simulink model "x35BusNetworkElectricityTransmissionModel"  (R2023b)
settings: Solver=VariableStepAuto  StartTime=0.0  StopTime=0.8  RelTol=1e-3
model workspace (MAT data in the model file):
  Compensation_Ki = 30
  Compensation_Kp = 3
  DC_Ki = 400
  DC_Kp = 8
  F = 0.01
  Flux_min = 0.5
  Grid_Freq_PWM = 2700
  Grid_Ireg_Ki = 5
  Grid_Ireg_Kp = 0.83
  Grid_Ireg_lim = 1.1
  Grid_Modindex_Upper = 1.1
  Grid_conv_Imax = 0.8
  H = 0.685
  Idref_max = 0.9
  Iqref_Tc = 0.3
  Ki_Var = 0.05
  Ki_Vreg = 20
  Ksh = 1.1
  L_pu = 0.3
  Llr = 0.16
  Lls = 0.18
  Lm = 2.9
  Nb_wt = 6
  P_mech = 1080000
  Pitch_Ki = 0
  Pitch_Kp = 150
  Pitch_Max = 27
  Pitch_Tc = 0.01
  Pitch_rate = 10
  Q_Filt = 50
  R_pu = 0.003
  Rotor_Freq_PWM = 1620
  Rotor_Ireg_Ki = 8
  Rotor_Ireg_Kp = 0.6
  Rotor_Ireg_lim = 0.1
  Rotor_Modindex_Upper = 2
  Rr = 0.016
  Rs = 0.023
  T_set = 0.0001
  Tp = 5e-05
  Ts = 5e-06
  Var_C_Filt = 720000
  Var_reg_max = 1.1
  Var_reg_min = 0.9
  WT_Coeff = [0.645 116 0.4 5 21 0.00912 0.08 0.035]
  WT_H = 4.32
  WT_IGBTRon = 5.931
  WT_Param = [91.204 10143]
  Wind_Freq_Filt = 10000
  Wind_Freq_nom = 60
  Wind_P_nom = 1200000
  Wind_Rotor_V_nom = 1950
  Wind_V_nom = 500
  Zeta_Filt = 0.707106781187
  init = [-0.2 0 0 0 0 0 0 0]
  p = 3
  torque0 = 0.83
  v_Ki = 0.1
  v_Kp = 3.6
  v_Max = 1.2
  v_Min = 0.7
  v_T = 5
  vreg_max = 1
  wind_VDC_nom = 1150
  wt0 = 1.2
undefined symbols (not defined in the file): D1, D11, Delta, DiscIntNeverNeededParam, Ion, Lithium, P, Q
libraries: powerlib_extras x144, spsSeriesRLCBranchLib x67, spsLoadFlowBusLib x43, spsThreePhaseTransformerTwoWindingsLib x32, spsThreePhaseSeriesRLCLoadLib x31, spsThreePhaseVIMeasurementLib x26, simulink_extras x26, spsDistributedParametersLineLib x22, spsGenericPowerSystemStabilizerLib x20, spsSynchronousMachinepuStandardLib x10, spsExcitationSystemLib x10, spsHydraulicTurbineandGovernorLib x10
(part 11 of 16)

== system x35BusNetworkElectricityTransmissionModel/ 41.4 MW Wind Generation/41.4 MW Wind Farm/Control System/Control System 3/Speed & Pitch Control System ==
  wr1 : Inport
  Meas_P : Inport  Port=2
  0-inf : Saturate  UpperLimit=inf  LowerLimit=0
  0-pitch_max : Saturate  UpperLimit=Pitch_Max  LowerLimit=0
  "0-pitch_max " : Saturate  UpperLimit=Pitch_Max  LowerLimit=0
  Constant2 : Constant
  Discrete PI Controller : Subsystem  DialogController=POWERSYS.PowerSysDialog  mask(Discrete PI Controller){Kp=v_Kp, Ki=v_Ki, Par_Limits=[vreg_max 0], Init=0.7, Ts=Ts}
      mask prompts: Kp "Proportional gain (Kp):"; Ki "Integral gain (Ki):"; Par_Limits "Output limits: [ Upper   Lower ]"; Init "Output initial value:"; Ts "Sample time:"
      mask help: This block implements a discrete PI controller.
      mask init:
      | UpperLimit=Par_Limits(1);
      | LowerLimit=Par_Limits(2);
      | power_initmask();
      mask Help: This block is part of a subset of blocks in the Extras library that does not have documentation associated with it, other than the block mask description.
      mask Display: disp('PI');
  Discrete PI Controller1 : powerlib_extras/Discrete  Control Blocks/Discrete PI Controller  Kp=Compensation_Kp  Ki=Compensation_Ki  Par_Limits=[Pitch_Max 0]  Init=0  Ts=Ts
  Gain2 : Gain  Gain=Pitch_Kp  SaturateOnIntegerOverflow=on  OutDataTypeStr=Inherit: Same as input  ParamDataTypeStr=Inherit: Same as input
  Rate Limiter   1 : RateLimiter  RisingSlewLimit=Pitch_rate  FallingSlewLimit=-Pitch_rate
  Saturation : Saturate  UpperLimit=v_Max  LowerLimit=v_Min
  Sum : Sum  Inputs=-+  SaturateOnIntegerOverflow=on
  Sum1 : Sum  Inputs=|+-
  Sum2 : Sum  Inputs=|+-  SaturateOnIntegerOverflow=on
  Sum3 : Sum  Inputs=|++
  Switch : Switch  Threshold=0.75  SaturateOnIntegerOverflow=off  InputSameDT=off
  Tracking Curve : Fcn  Expr=-0.67*u(1)^2+1.42*u(1)+0.51
  pu_elec->pu_mec : Gain  Gain=Wind_P_nom/P_mech
  t=Pitch_time_constant : powerlib_extras/Discrete  Control Blocks/Discrete 1st-Order Filter  FilterType=Lowpass  Tc=Pitch_Tc  Ts=Ts  Initialize=on  Vac_Init=[0.8 -25 60]*0  Vdc_Init=0  PlotResponse=off  param1=[1 500 0.1]
  t=T_speed : powerlib_extras/Discrete  Control Blocks/Discrete 1st-Order Filter  FilterType=Lowpass  Tc=v_T  Ts=Ts  Initialize=on  Vac_Init=[0 0 0]  Vdc_Init=1-init(1)  PlotResponse=off  param1=[1 500 0.1]
  wref : Constant  Value=1.2
  Tem_cmd : Outport  VectorParamsAs1DForOutWhenUnconnected=off
  Pitch (deg) : Outport  Port=2  VectorParamsAs1DForOutWhenUnconnected=off
  wires:
  Rate Limiter   1/1 -> "0-pitch_max "/1
  Switch/1 -> Saturation/1
  Sum3/1 -> Rate Limiter   1/1
  Sum1/1 -> Discrete PI Controller/1(Error)
  Saturation/1 -> t=T_speed/1
  Constant2/1 -> Sum2/2  "Pref"
  Discrete PI Controller1/1 -> Sum3/2
  Meas_P/1 -> 0-inf/1
  t=T_speed/1 -> Sum/1, Sum1/2  "wref"
  0-inf/1 -> pu_elec->pu_mec/1
  wr1/1 -> Sum/2, Sum1/1
  wref/1 -> Switch/1
  0-pitch_max/1 -> Sum3/1
  Discrete PI Controller/1(Out) -> Tem_cmd/1
  t=Pitch_time_constant/1 -> Pitch (deg)/1
  Sum2/1 -> Discrete PI Controller1/1
  Gain2/1 -> 0-pitch_max/1
  pu_elec->pu_mec/1 -> Switch/2, Tracking Curve/1, Sum2/1
  "0-pitch_max "/1 -> t=Pitch_time_constant/1
  Sum/1 -> Gain2/1
  Tracking Curve/1 -> Switch/3

== system x35BusNetworkElectricityTransmissionModel/ 41.4 MW Wind Generation/41.4 MW Wind Farm/Control System/Control System 4/Grid-side Control System ==
  note: Required value for modulation index "m" to obtain 1 pu generated voltage by the converter:
  note: m = Vnom * 2*sqrt(2/3) / Vdc
  note: Where Vnom = RMS ph-ph nominal voltage
  Stator_Vdq : Inport
  Iq_ref : Inport  Port=2
  Vdc : Inport  Port=3
  Grid_conv_Idq : Inport  Port=4
  Theta_PLL : Inport  Port=5
  w : Inport  Port=6
  Current Regulator : Subsystem
  Grid Voltage Converter : Subsystem
  Modulation : Subsystem
  VDC Regulator : Subsystem
  Grid_conv_V : Outport  VectorParamsAs1DForOutWhenUnconnected=off
  wires:
  Current Regulator/1(Grid_conv_Vd) -> Modulation/1(x)
  Current Regulator/2(Grid_conv_Vq) -> Modulation/2(y)
  Grid Voltage Converter/1(Grid_conv_V) -> Grid_conv_V/1
  Theta_PLL/1 -> Grid Voltage Converter/2(Theta_PLL)
  VDC Regulator/1(Out1) -> Current Regulator/2(In2)
  Iq_ref/1 -> VDC Regulator/1(Iq_ref)
  Grid_conv_Idq/1 -> Current Regulator/3(Grid_conv_Idq)
  Stator_Vdq/1 -> Current Regulator/1(Stator_Vdq)
  w/1 -> Current Regulator/4(w)
  Modulation/1(Vdq0) -> Grid Voltage Converter/1(dq0)
  Vdc/1 -> VDC Regulator/2(Vdc)

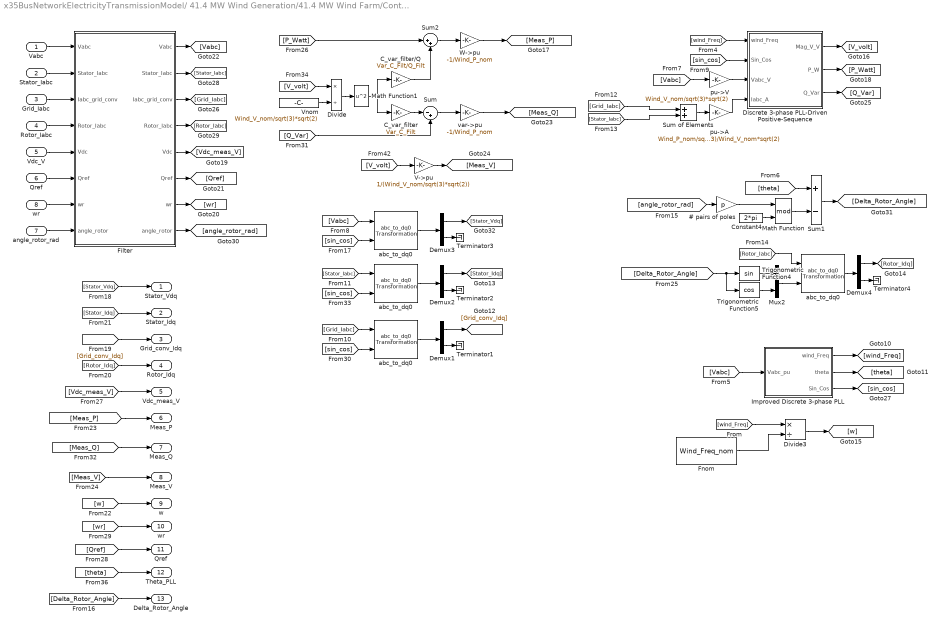
== system x35BusNetworkElectricityTransmissionModel/ 41.4 MW Wind Generation/41.4 MW Wind Farm/Control System/Control System 4/Measurement and abc-to-dq transformation  ==
  Vabc : Inport
  Stator_Iabc : Inport  Port=2
  Grid_Iabc : Inport  Port=3
  Rotor_Iabc : Inport  Port=4
  Vdc_V : Inport  Port=5
  Qref : Inport  Port=6
  angle_rotor_rad : Inport  Port=7
  wr : Inport  Port=8
  "   abc_to_dq0    " : powerlib_extras/Measurements/abc_to_dq0 Transformation
  " Improved Discrete 3-phase PLL" : Subsystem  mask(Discrete 3-phase PLL){Fmin=0.75*Wind_Freq_nom, Par_Init=[0 Wind_Freq_nom], ParK=[5 3.2 1 50], Ts=Ts}
      mask prompts: Fmin "Minimum frequency (Hz):"; Par_Init "Initial inputs:[ Phase(degrees)   Frequency(Hz) ]"; ParK "Regulator gains [ Kp1 Kp2  Ki1  Ki2 ]"; Ts "Sample time:"
      mask help:
      | This Phase Locked Loop (PLL) system can be used  to synchronize on a set of variable frequency, three-phase sinusoidal signals.
      |
      | Input 1: Vector containing the normalized
      |              three-phase signals [Va Vb Vc]
      | Output 1:  Measured frequency (Hz) = w/(2pi)
      | Output 2:  Ramp w.t   varying between  0 and 2*pi,
      | synchronized on zero crossings of the fundamental (positive-sequence) of phase A.
      | Output 3: Vector [sin(wt) cos(wt)]
      mask init:
      | Kp1=ParK(1);
      | Kp2=ParK(2);
      | Ki1=ParK(3);
      | Ki2=ParK(4);
      | Phase_Init=Par_Init(1);
      | Finit=Par_Init(2);
      | power_initmask();
      settings: OpenFcn=power_openblockproxy();
  # pairs of poles : Gain  Gain=p  SaturateOnIntegerOverflow=on  OutDataTypeStr=Inherit: Same as input  ParamDataTypeStr=Inherit: Same as input
  C_var_filter : Gain  Gain=Var_C_Filt  SaturateOnIntegerOverflow=on  OutDataTypeStr=Inherit: Same as input  ParamDataTypeStr=Inherit: Same as input
  C_var_filter/Q : Gain  Gain=Var_C_Filt/Q_Filt  SaturateOnIntegerOverflow=on  OutDataTypeStr=Inherit: Same as input  ParamDataTypeStr=Inherit: Same as input
  Constant4 : Constant  Value=2*pi
  Demux{1..4} (4 alike) : Demux  Outputs=[2 1]
      settings: DisplayOption=none
  "Discrete 3-phase PLL-Driven Positive-Sequence " : Subsystem  mask(Discrete 3-phase PLL-Driven Positive-Sequence Active & Reactive Power){Finit=Wind_Freq_nom, Fmin=Wind_Freq_nom*45/60, Par_Vinit=[Wind_V_nom/sqrt(3)*sqrt(2) 30], Par_Iinit=[Wind_P_nom/sqrt(3)/Wind_V_nom*sqrt(2) -10], Ts=Ts}
      mask prompts: Finit "Initial frequency (Hz):"; Fmin "Minimum frequency (Hz):"; Par_Vinit "Voltage initial input: [ Mag  Phase(Degrees) ]"; Par_Iinit "Current initial input: [ Mag  Phase(Degrees) ]"; Ts "Sample time:"
      mask help:
      | This discrete block measures the 3-phase active power P and reactive power Q  associated with a periodic set of 3-phase voltages and currents which may contain harmonics. P and Q are calculated by evaluating the fundamental values (positive-sequence) of the input voltages and currents with a running window over one cycle of the specified frequency (port Freq).
      |  Input port "Sin_Cos" (a two-dimension signal) provides the reference frame required for the computation.
      |
      | input 1: must give the frequency of the fundamental (Hz)
      | Input 2: must contain a  [sin(wt)  cos(wt)] two dimension signal , where w is the rotation speed (rad/s) of the reference frame used for the computation..
      | input 3: Vectorized 3-phase  instantaneous voltage (Vabc)
      | input 4: Vectorized 3-phase instantaneous current (Iabc)
      |
      | Output 1: Vector [Mag_V Mag_I] of the fundamental values (Magnitude) of the voltage & current (peak values of the positive-sequence)
      | Output 2: 3-phase PQ measurement vector [P(W) Q (var)] evaluated at the specified frequency. Current flowing into an RL circuit will produce  positive active and reactive powers.
      |
      | For the first cycle of simulation, the outputs are held constant using the values specified by the parameters "Initial input".
      | he value of the parameter "Minimum frequency" is used to determine the buffer size of the "Variable Transport Delay" block found inside this subsystem.
      mask init:
      | power_initmask();
      settings: OpenFcn=power_openblockproxy();
  Divide : Product  Inputs=*/
  Divide3 : Product  Inputs=*/
  Filter : Subsystem  mask{Freq=Wind_Freq_Filt, Zeta1=Zeta_Filt, Ts=Ts}
      mask prompts: Freq "Cut-off frequency (Hz):"; Zeta1 "Damping factor Zeta:"; Ts "Sample time"
  Fnom : Constant  Value=Wind_Freq_nom
  Math Function : Math  Operator=mod  SignedPower=on
  Math Function1 : Math  Operator=square  SignedPower=on
  Mux2 : Mux  Inputs=2
  Sum : Sum  Inputs=|-+
  Sum of Elements : Sum
  Sum1 : Sum  Inputs=+-  InputSameDT=on  SaturateOnIntegerOverflow=on  OutDataTypeStr=Inherit: Same as first input
  Sum2 : Sum  Inputs=|++
  Terminator{1..4} (4 alike) : Terminator
  Trigonometric Function4 : Trigonometry
  Trigonometric Function5 : Trigonometry  Operator=cos
  V->pu : Gain  Gain=1/(Wind_V_nom/sqrt(3)*sqrt(2))  SaturateOnIntegerOverflow=on  OutDataTypeStr=Inherit: Same as input  ParamDataTypeStr=Inherit: Same as input
  Vnom : Constant  Value=Wind_V_nom/sqrt(3)*sqrt(2)
  W->pu : Gain  Gain=-1/Wind_P_nom  SaturateOnIntegerOverflow=on  OutDataTypeStr=Inherit: Same as input  ParamDataTypeStr=Inherit: Same as input
  abc_to_dq0 : powerlib_extras/Measurements/abc_to_dq0 Transformation
  "abc_to_dq0 " : powerlib_extras/Measurements/abc_to_dq0 Transformation
  "abc_to_dq0  " : powerlib_extras/Measurements/abc_to_dq0 Transformation
  pu->A : Gain  Gain=Wind_P_nom/sqrt(3)/Wind_V_nom*sqrt(2)  SaturateOnIntegerOverflow=on  OutDataTypeStr=Inherit: Same as input  ParamDataTypeStr=Inherit: Same as input
  pu->V : Gain  Gain=Wind_V_nom/sqrt(3)*sqrt(2)  SaturateOnIntegerOverflow=on  OutDataTypeStr=Inherit: Same as input  ParamDataTypeStr=Inherit: Same as input
  "var->pu " : Gain  Gain=-1/Wind_P_nom  SaturateOnIntegerOverflow=on  OutDataTypeStr=Inherit: Same as input  ParamDataTypeStr=Inherit: Same as input
  Stator_Vdq : Outport  VectorParamsAs1DForOutWhenUnconnected=off
  Stator_Idq : Outport  Port=2  VectorParamsAs1DForOutWhenUnconnected=off
  Grid_conv_Idq : Outport  Port=3  VectorParamsAs1DForOutWhenUnconnected=off
  Rotor_Idq : Outport  Port=4  VectorParamsAs1DForOutWhenUnconnected=off
  Vdc_meas_V : Outport  Port=5  VectorParamsAs1DForOutWhenUnconnected=off
  Meas_P : Outport  Port=6  VectorParamsAs1DForOutWhenUnconnected=off
  Meas_Q : Outport  Port=7  VectorParamsAs1DForOutWhenUnconnected=off
  Meas_V : Outport  Port=8  VectorParamsAs1DForOutWhenUnconnected=off
  w : Outport  Port=9  VectorParamsAs1DForOutWhenUnconnected=off
  "wr " : Outport  Port=10  VectorParamsAs1DForOutWhenUnconnected=off
  "Qref " : Outport  Port=11  VectorParamsAs1DForOutWhenUnconnected=off
  Theta_PLL : Outport  Port=12  VectorParamsAs1DForOutWhenUnconnected=off
  Delta_Rotor_Angle : Outport  Port=13  VectorParamsAs1DForOutWhenUnconnected=off
  wires:
  Math Function/1 -> Sum1/2
  [wind_Freq] -> "Discrete 3-phase PLL-Driven Positive-Sequence "/1(wind_Freq)
  [P_Watt] -> Sum2/1
  [sin_cos] -> abc_to_dq0/2
  [Meas_Q] -> Meas_Q/1
  [Q_Var] -> Sum/2
  Math Function1/1 -> C_var_filter/Q/1, C_var_filter/1
  Sum of Elements/1 -> pu->A/1
  [Grid_Iabc] -> Sum of Elements/1
  [Grid_conv_Idq] -> Grid_conv_Idq/1
  Filter/6("Qref ") -> [Qref]
  W->pu/1 -> [Meas_P]
  [Stator_Idq] -> Stator_Idq/1
  "Discrete 3-phase PLL-Driven Positive-Sequence "/1(Mag_V_V) -> [V_volt]
  Demux1/2 -> Terminator1/1
  [wr] -> "wr "/1
  Filter/3("Iabc_grid_conv ") -> [Grid_Iabc]
  Filter/2("Stator_Iabc ") -> [Stator_Iabc]
  [Meas_P] -> Meas_P/1
  [Delta_Rotor_Angle] -> Trigonometric Function4/1, Trigonometric Function5/1
  Vnom/1 -> Divide/2
  [w] -> w/1
  "var->pu "/1 -> [Meas_Q]
  Sum2/1 -> W->pu/1
  [wind_Freq] -> Divide3/1
  [Delta_Rotor_Angle] -> Delta_Rotor_Angle/1
  Vdc_V/1 -> Filter/5(Vdc)
  "Discrete 3-phase PLL-Driven Positive-Sequence "/3(Q_Var) -> [Q_Var]
  [Vabc] -> pu->V/1
  wr/1 -> Filter/7(wr)
  Fnom/1 -> Divide3/2
  [Vabc] -> " Improved Discrete 3-phase PLL"/1(Vabc_pu)
  "Discrete 3-phase PLL-Driven Positive-Sequence "/2(P_W) -> [P_Watt]
  Trigonometric Function5/1 -> Mux2/2
  [sin_cos] -> "abc_to_dq0 "/2
  [V_volt] -> Divide/1
  Demux3/2 -> Terminator3/1
  Filter/5("Vdc ") -> [Vdc_meas_V]
  Filter/1("Vabc ") -> [Vabc]
  [sin_cos] -> "abc_to_dq0  "/2
  angle_rotor_rad/1 -> Filter/8(angle_rotor)
  "   abc_to_dq0    "/1 -> Demux4/1
  Divide3/1 -> [w]
  Divide/1 -> Math Function1/1
  # pairs of poles/1 -> Math Function/1
  [Stator_Iabc] -> "abc_to_dq0 "/1
  Filter/8("angle_rotor ") -> [angle_rotor_rad]
  Sum/1 -> "var->pu "/1
  [Stator_Vdq] -> Stator_Vdq/1
  Demux4/1 -> [Rotor_Idq]
  [Grid_Iabc] -> "abc_to_dq0  "/1
  [angle_rotor_rad] -> # pairs of poles/1
  Mux2/1 -> "   abc_to_dq0    "/2
  Demux2/2 -> Terminator2/1
  [V_volt] -> V->pu/1
  [Rotor_Iabc] -> "   abc_to_dq0    "/1
  Demux1/1 -> [Grid_conv_Idq]
  Filter/7("wr ") -> [wr]
  [Meas_V] -> Meas_V/1
  [Rotor_Idq] -> Rotor_Idq/1
  Constant4/1 -> Math Function/2
  Demux4/2 -> Terminator4/1
  [sin_cos] -> "Discrete 3-phase PLL-Driven Positive-Sequence "/2(Sin_Cos)
  Qref/1 -> Filter/6(Qref)
  Trigonometric Function4/1 -> Mux2/1
  [Vabc] -> abc_to_dq0/1
  Vabc/1 -> Filter/1(Vabc)
  Rotor_Iabc/1 -> Filter/4(Rotor_Iabc)
  [Qref] -> "Qref "/1
  C_var_filter/Q/1 -> Sum2/2
  Grid_Iabc/1 -> Filter/3(Iabc_grid_conv)
  " Improved Discrete 3-phase PLL"/3(Sin_Cos) -> [sin_cos]
  abc_to_dq0/1 -> Demux3/1
  Stator_Iabc/1 -> Filter/2(Stator_Iabc)
  V->pu/1 -> [Meas_V]
  "abc_to_dq0  "/1 -> Demux1/1
  Demux3/1 -> [Stator_Vdq]
  " Improved Discrete 3-phase PLL"/1(wind_Freq) -> [wind_Freq]
  [theta] -> Theta_PLL/1
  [Vdc_meas_V] -> Vdc_meas_V/1
  Filter/4("Rotor_Iabc ") -> [Rotor_Iabc]
  Sum1/1 -> [Delta_Rotor_Angle]
  "abc_to_dq0 "/1 -> Demux2/1
  [Stator_Iabc] -> Sum of Elements/2
  C_var_filter/1 -> Sum/1
  pu->V/1 -> "Discrete 3-phase PLL-Driven Positive-Sequence "/3(Vabc_V)
  Demux2/1 -> [Stator_Idq]
  [theta] -> Sum1/1
  " Improved Discrete 3-phase PLL"/2(theta) -> [theta]
  pu->A/1 -> "Discrete 3-phase PLL-Driven Positive-Sequence "/4(Iabc_A)

== system x35BusNetworkElectricityTransmissionModel/ 41.4 MW Wind Generation/41.4 MW Wind Farm/Control System/Control System 4/Rotor-side Control System ==
  Rotor_Idq : Inport
  wr : Inport  Port=2
  Vdc : Inport  Port=3
  Angle : Inport  Port=4
  Qref : Inport  Port=5
  Meas_Q : Inport  Port=6
  Meas_V : Inport  Port=7
  Stator_Vdq : Inport  Port=8
  w : Inport  Port=9
  Stator_Idq : Inport  Port=10
  Tem_cmd : Inport  Port=11
  Current Regulator : Subsystem
  "Electromagnetic Torque Controller " : Subsystem
  Gain : Gain  Gain=-1
  "Iqr, ref_limit" : Subsystem
  Modulation Index & Phase : Subsystem
  Rotor Control Voltage Converter : Subsystem
  Var Regulator : Subsystem
  Voltage Regulator : Subsystem
  Uctrl_rotor_conv : Outport  VectorParamsAs1DForOutWhenUnconnected=off
  wires:
  "Electromagnetic Torque Controller "/1(Rotor_Id_ref) -> Current Regulator/1(Rotor_Id_ref), "Iqr, ref_limit"/1(Rotor_Id_ref)
  Qref/1 -> Var Regulator/1(Qref)
  Meas_Q/1 -> Var Regulator/2(Meas_Q)
  Meas_V/1 -> Var Regulator/3(Meas_V)
  "Iqr, ref_limit"/1(Iqrlim) -> Voltage Regulator/1(Max), Gain/1
  Var Regulator/1(Out1) -> Voltage Regulator/3(In)
  Rotor_Idq/1 -> Current Regulator/2(Rotor_Idq)
  wr/1 -> Current Regulator/4(wr)
  Voltage Regulator/1(Iqr_ref) -> Current Regulator/3(Iqr_ref)
  Angle/1 -> Rotor Control Voltage Converter/3(Angle)
  Rotor Control Voltage Converter/1(Uctrl_rotor_conv) -> Uctrl_rotor_conv/1
  Vdc/1 -> Modulation Index & Phase/3(Vdc)
  Modulation Index & Phase/1(x1) -> Rotor Control Voltage Converter/1(x1)
  Modulation Index & Phase/2(y1) -> Rotor Control Voltage Converter/2(y1)
  Current Regulator/1(Rotor_conv_Vd) -> Modulation Index & Phase/1(x)
  Current Regulator/2(Rotor_conv_Vq) -> Modulation Index & Phase/2(y)
  Stator_Vdq/1 -> "Electromagnetic Torque Controller "/1(Stator_Vdq)
  w/1 -> "Electromagnetic Torque Controller "/2(w)
  Stator_Idq/1 -> "Electromagnetic Torque Controller "/3(Stator_Idq)
  Tem_cmd/1 -> "Electromagnetic Torque Controller "/4(Tem_cmd)
  Gain/1 -> Voltage Regulator/2(Min)

== system x35BusNetworkElectricityTransmissionModel/ 41.4 MW Wind Generation/41.4 MW Wind Farm/Control System/Control System 4/Speed & Pitch Control System ==
  wr1 : Inport
  Meas_P : Inport  Port=2
  0-inf : Saturate  UpperLimit=inf  LowerLimit=0
  0-pitch_max : Saturate  UpperLimit=Pitch_Max  LowerLimit=0
  "0-pitch_max " : Saturate  UpperLimit=Pitch_Max  LowerLimit=0
  Constant2 : Constant
  Discrete PI Controller : Subsystem  DialogController=POWERSYS.PowerSysDialog  mask(Discrete PI Controller){Kp=v_Kp, Ki=v_Ki, Par_Limits=[vreg_max 0], Init=0.7, Ts=Ts}
      mask prompts: Kp "Proportional gain (Kp):"; Ki "Integral gain (Ki):"; Par_Limits "Output limits: [ Upper   Lower ]"; Init "Output initial value:"; Ts "Sample time:"
      mask help: This block implements a discrete PI controller.
      mask init:
      | UpperLimit=Par_Limits(1);
      | LowerLimit=Par_Limits(2);
      | power_initmask();
      mask Help: This block is part of a subset of blocks in the Extras library that does not have documentation associated with it, other than the block mask description.
      mask Display: disp('PI');
  Discrete PI Controller1 : powerlib_extras/Discrete  Control Blocks/Discrete PI Controller  Kp=Compensation_Kp  Ki=Compensation_Ki  Par_Limits=[Pitch_Max 0]  Init=0  Ts=Ts
  Gain2 : Gain  Gain=Pitch_Kp  SaturateOnIntegerOverflow=on  OutDataTypeStr=Inherit: Same as input  ParamDataTypeStr=Inherit: Same as input
  Rate Limiter   1 : RateLimiter  RisingSlewLimit=Pitch_rate  FallingSlewLimit=-Pitch_rate
  Saturation : Saturate  UpperLimit=v_Max  LowerLimit=v_Min
  Sum : Sum  Inputs=-+  SaturateOnIntegerOverflow=on
  Sum1 : Sum  Inputs=|+-
  Sum2 : Sum  Inputs=|+-  SaturateOnIntegerOverflow=on
  Sum3 : Sum  Inputs=|++
  Switch : Switch  Threshold=0.75  SaturateOnIntegerOverflow=off  InputSameDT=off
  Tracking Curve : Fcn  Expr=-0.67*u(1)^2+1.42*u(1)+0.51
  pu_elec->pu_mec : Gain  Gain=Wind_P_nom/P_mech
  t=Pitch_time_constant : powerlib_extras/Discrete  Control Blocks/Discrete 1st-Order Filter  FilterType=Lowpass  Tc=Pitch_Tc  Ts=Ts  Initialize=on  Vac_Init=[0.8 -25 60]*0  Vdc_Init=0  PlotResponse=off  param1=[1 500 0.1]
  t=T_speed : powerlib_extras/Discrete  Control Blocks/Discrete 1st-Order Filter  FilterType=Lowpass  Tc=v_T  Ts=Ts  Initialize=on  Vac_Init=[0 0 0]  Vdc_Init=1-init(1)  PlotResponse=off  param1=[1 500 0.1]
  wref : Constant  Value=1.2
  Tem_cmd : Outport  VectorParamsAs1DForOutWhenUnconnected=off
  Pitch (deg) : Outport  Port=2  VectorParamsAs1DForOutWhenUnconnected=off
  wires:
  Rate Limiter   1/1 -> "0-pitch_max "/1
  Switch/1 -> Saturation/1
  Sum3/1 -> Rate Limiter   1/1
  Sum1/1 -> Discrete PI Controller/1(Error)
  Saturation/1 -> t=T_speed/1
  Constant2/1 -> Sum2/2  "Pref"
  Discrete PI Controller1/1 -> Sum3/2
  Meas_P/1 -> 0-inf/1
  t=T_speed/1 -> Sum/1, Sum1/2  "wref"
  0-inf/1 -> pu_elec->pu_mec/1
  wr1/1 -> Sum/2, Sum1/1
  wref/1 -> Switch/1
  0-pitch_max/1 -> Sum3/1
  Discrete PI Controller/1(Out) -> Tem_cmd/1
  t=Pitch_time_constant/1 -> Pitch (deg)/1
  Sum2/1 -> Discrete PI Controller1/1
  Gain2/1 -> 0-pitch_max/1
  pu_elec->pu_mec/1 -> Switch/2, Tracking Curve/1, Sum2/1
  "0-pitch_max "/1 -> t=Pitch_time_constant/1
  Sum/1 -> Gain2/1
  Tracking Curve/1 -> Switch/3

== system x35BusNetworkElectricityTransmissionModel/ 41.4 MW Wind Generation/41.4 MW Wind Farm/Control System/Control System 1/Grid-side Control System/Current Regulator ==
  Stator_Vdq : Inport
  In2 : Inport  Port=2
  Grid_conv_Idq : Inport  Port=3
  w : Inport  Port=4
  Constant1 : Constant  Value=L_pu
  Constant2 : Constant  Value=L_pu
  Constant3 : Constant  Value=R_pu
  Constant4 : Constant  Value=R_pu
  Demux{,1..3} (4 alike) : Demux  Outputs=2
      settings: DisplayOption=none
  Discrete PI Controller1 : powerlib_extras/Discrete  Control Blocks/Discrete PI Controller  Kp=Grid_Ireg_Kp  Ki=Grid_Ireg_Ki  Par_Limits=[1.0 -1.0] *Grid_Ireg_lim  Init=0  Ts=Ts
  Mux2 : Mux  Inputs=2
  Product : Product  Inputs=3  InputSameDT=on  SaturateOnIntegerOverflow=on  OutDataTypeStr=Inherit: Same as first input
  Product1 : Product  Inputs=3  InputSameDT=on  SaturateOnIntegerOverflow=on  OutDataTypeStr=Inherit: Same as first input
  Product2 : Product  InputSameDT=on  SaturateOnIntegerOverflow=on  OutDataTypeStr=Inherit: Same as first input
  Product3 : Product  InputSameDT=on  SaturateOnIntegerOverflow=on  OutDataTypeStr=Inherit: Same as first input
  Sum1 : Sum  Inputs=+-  InputSameDT=on  SaturateOnIntegerOverflow=on  OutDataTypeStr=Inherit: Same as first input
  Sum2 : Sum  Inputs=-+|  InputSameDT=on  SaturateOnIntegerOverflow=on  OutDataTypeStr=Inherit: Same as first input
  Sum3 : Sum  Inputs=||++-  InputSameDT=on  SaturateOnIntegerOverflow=on  OutDataTypeStr=Inherit: Same as first input
  Sum4 : Sum  Inputs=|+-  InputSameDT=on  SaturateOnIntegerOverflow=on  OutDataTypeStr=Inherit: Same as first input
  Sum5 : Sum  Inputs=|--+  InputSameDT=on  SaturateOnIntegerOverflow=on  OutDataTypeStr=Inherit: Same as first input
  Sum6 : Sum  Inputs=|-+  InputSameDT=on  SaturateOnIntegerOverflow=on  OutDataTypeStr=Inherit: Same as first input
  Grid_conv_Vd : Outport
  Grid_conv_Vq : Outport  Port=2
  wires:
  Product1/1 -> Sum5/2
  Product2/1 -> Sum3/3
  Product3/1 -> Sum5/1
  [id_ref] -> Product2/2
  Sum1/1 -> Grid_conv_Vd/1  "Grid_conv_Vd"
  Demux1/2 -> [iq_ref], Sum2/2  "Iq_ref"
  Demux/1 -> Sum4/2  "Id"
  [w] -> Product/2
  Demux2/2 -> Sum5/3  "Vq"
  [iq_ref] -> Product/3
  Sum4/1 -> Mux2/1
  Constant4/1 -> Product3/2
  Stator_Vdq/1 -> Demux2/1
  Constant2/1 -> Product1/2
  Constant3/1 -> Product2/1
  Grid_conv_Idq/1 -> Demux/1
  Product/1 -> Sum3/2
  Discrete PI Controller1/1 -> Demux3/1
  Sum2/1 -> Mux2/2
  Sum6/1 -> Grid_conv_Vq/1  "Grid_conv_Vq"
  w/1 -> [w]
  [id_ref] -> Product1/1
  Sum5/1 -> Sum6/2
  [iq_ref] -> Product3/1
  Sum3/1 -> Sum1/1
  Mux2/1 -> Discrete PI Controller1/1
  Demux2/1 -> Sum3/1  "Vd"
  Demux1/1 -> Sum4/1, [id_ref]  "Id_ref"
  Demux3/1 -> Sum1/2  "vd'"
  Constant1/1 -> Product/1
  Demux/2 -> Sum2/1  "Iq"
  Demux3/2 -> Sum6/1  "vq'"
  [w] -> Product1/3
  In2/1 -> Demux1/1

== system x35BusNetworkElectricityTransmissionModel/ 41.4 MW Wind Generation/41.4 MW Wind Farm/Control System/Control System 1/Grid-side Control System/Grid Voltage Converter ==
  dq0 : Inport
  Theta_PLL : Inport  Port=2
  Mux5 : Mux  Inputs=2
  Trigonometric Function2 : Trigonometry
  Trigonometric Function3 : Trigonometry  Operator=cos
  dq0_to_abc Transformation : powerlib_extras/Measurements/dq0_to_abc Transformation
  Grid_conv_V : Outport  VectorParamsAs1DForOutWhenUnconnected=off
  wires:
  Trigonometric Function2/1 -> Mux5/1
  Mux5/1 -> dq0_to_abc Transformation/2
  Theta_PLL/1 -> Trigonometric Function2/1, Trigonometric Function3/1
  dq0_to_abc Transformation/1 -> Grid_conv_V/1
  dq0/1 -> dq0_to_abc Transformation/1
  Trigonometric Function3/1 -> Mux5/2

== system x35BusNetworkElectricityTransmissionModel/ 41.4 MW Wind Generation/41.4 MW Wind Farm/Control System/Control System 1/Grid-side Control System/Modulation ==
  x : Inport
  y : Inport  Port=2
  1 : Saturate  UpperLimit=Grid_Modindex_Upper  LowerLimit=0
  Avoid division by zero : Saturate  UpperLimit=inf  LowerLimit=1e-6
  Cartesian to Polar1 : simulink_extras/Transformations/Cartesian to Polar
  K : Constant  Value=Wind_V_nom*2*sqrt(2/3)
  Mux4 : Mux  Inputs=3
  Polar to Cartesian : simulink_extras/Transformations/Polar to Cartesian
  Product4 : Product  Inputs=**/  InputSameDT=on  SaturateOnIntegerOverflow=on  OutDataTypeStr=Inherit: Same as first input
  V0 : Constant  Value=0
  Vdq0 : Outport
  wires:
  K/1 -> Product4/2
  Polar to Cartesian/2 -> Mux4/2
  V0/1 -> Mux4/3
  y/1 -> Cartesian to Polar1/2
  [Vdc] -> Avoid division by zero/1
  Polar to Cartesian/1 -> Mux4/1
  Mux4/1 -> Vdq0/1  "Vdq0"
  Avoid division by zero/1 -> Product4/3
  1/1 -> Polar to Cartesian/1
  Cartesian to Polar1/2 -> Polar to Cartesian/2
  Product4/1 -> 1/1  "m"
  x/1 -> Cartesian to Polar1/1
  Cartesian to Polar1/1 -> Product4/1

== system x35BusNetworkElectricityTransmissionModel/ 41.4 MW Wind Generation/41.4 MW Wind Farm/Control System/Control System 1/Grid-side Control System/VDC Regulator ==
  Iq_ref : Inport
  Vdc : Inport  Port=2
  ->pu : Gain  Gain=1/wind_VDC_nom
  Discrete PI Controller : powerlib_extras/Discrete  Control Blocks/Discrete PI Controller  Kp=DC_Kp  Ki=DC_Ki  Par_Limits=[1 -1]*Grid_conv_Imax  Init=0  Ts=Ts
  Mux : Mux  Inputs=2
  Sum7 : Sum  Inputs=|+-  InputSameDT=on  SaturateOnIntegerOverflow=on  OutDataTypeStr=Inherit: Same as first input
  Vdc_ref (V) : Constant  Value=wind_VDC_nom
  Out1 : Outport
  wires:
  Vdc/1 -> [Vdc], Sum7/2
  Iq_ref/1 -> Mux/2
  Mux/1 -> Out1/1
  Discrete PI Controller/1 -> Mux/1  "Id_ref"
  ->pu/1 -> Discrete PI Controller/1
  Vdc_ref (V)/1 -> Sum7/1
  Sum7/1 -> ->pu/1

== system x35BusNetworkElectricityTransmissionModel/ 41.4 MW Wind Generation/41.4 MW Wind Farm/Control System/Control System 1/Measurement and abc-to-dq transformation / Improved Discrete 3-phase PLL ==
  note: Pierre Giroux, Gilbert Sybille, R. Gagnon
      | Power System Laboratory, IREQ
      | Hydro-Quebec
  note: New Discrete 3-phase PLL
  Vabc_pu : Inport  PortDimensions=3
  2nd-Order Filter : powerlib_extras/Discrete  Control Blocks/Discrete  2nd-Order Filter  FilterType=Lowpass  Fo=25  Zeta=0.707  Ts=Ts  Initialize=on  Vac_Init=[0 0 Finit]  Vdc_Init=Finit  PlotResponse=off  param1=[1 500 0.1]
  Constant1 : Constant  Value=2*pi*Finit
  Constant4 : Constant  Value=2*pi
  Discrete-Time Integrator : DiscreteIntegrator  SampleTime=Ts  ICPrevOutput=DiscIntNeverNeededParam  ICPrevScaledInput=DiscIntNeverNeededParam
  Discrete-Time Integrator1 : DiscreteIntegrator  gainval=1  SampleTime=Ts  LimitOutput=on  UpperSaturationLimit=2*pi*5  LowerSaturationLimit=-2*pi*5  ICPrevOutput=DiscIntNeverNeededParam  ICPrevScaledInput=DiscIntNeverNeededParam
  Gain10 : Gain  Gain=1/2/pi  SaturateOnIntegerOverflow=on  OutDataTypeStr=Inherit: Same as input  ParamDataTypeStr=Inherit: Same as input
  Kp1 : Gain  Gain=Kp2  SaturateOnIntegerOverflow=on  OutDataTypeStr=Inherit: Same as input  ParamDataTypeStr=Inherit: Same as input
  Kp2 : Gain  Gain=Ki2  SaturateOnIntegerOverflow=on  OutDataTypeStr=Inherit: Same as input  ParamDataTypeStr=Inherit: Same as input
  Kp3 : Gain  Gain=Ki1  SaturateOnIntegerOverflow=on  OutDataTypeStr=Inherit: Same as input  ParamDataTypeStr=Inherit: Same as input
  Kp4 : Gain  Gain=Kp1  SaturateOnIntegerOverflow=on  OutDataTypeStr=Inherit: Same as input  ParamDataTypeStr=Inherit: Same as input
  Math Function : Math  Operator=mod  SignedPower=on
  Mux2 : Mux  Inputs=2
  Rate Limiter : powerlib_extras/Discrete  Control Blocks/Discrete Rate Limiter  R=12  F=-12  Vinit=Finit  Ts=Ts
  Selector : Selector  InputPortWidth=3  IndexOptions=Index vector (dialog)  Indices=2  OutputSizes=1
  Sum : Sum  Inputs=+++
  Trigonometric Function : Trigonometry
  Trigonometric Function1 : Trigonometry  Operator=atan
  Trigonometric Function2 : Trigonometry  Operator=cos
  Trigonometric Function3 : Trigonometry  Operator=atan
  Unit Delay : UnitDelay  InitialCondition=Finit  SampleTime=Ts  HasFrameUpgradeWarning=on
  Variable Frequency Mean value : powerlib_extras/Discrete Measurements/Discrete Variable Frequency Mean value  Finit=Finit  Fmin=Fmin  Vinit=0  Ts=Ts
  abc_to_dq0 Transformation : powerlib_extras/Measurements/abc_to_dq0 Transformation
  wind_Freq : Outport  VectorParamsAs1DForOutWhenUnconnected=off
  theta : Outport  Port=2  VectorParamsAs1DForOutWhenUnconnected=off
  Sin_Cos : Outport  Port=3  VectorParamsAs1DForOutWhenUnconnected=off
  wires:
  Discrete-Time Integrator1/1 -> Sum/2
  Kp1/1 -> Sum/1
  Discrete-Time Integrator/1 -> Math Function/1
  Unit Delay/1 -> Variable Frequency Mean value/1, wind_Freq/1
  Sum/1 -> Gain10/1, Discrete-Time Integrator/1
  Kp2/1 -> Discrete-Time Integrator1/1
  Trigonometric Function3/1 -> Kp2/1
  Kp3/1 -> Trigonometric Function3/1
  Variable Frequency Mean value/1 -> Kp3/1, Kp4/1
  Constant1/1 -> Sum/3
  Trigonometric Function1/1 -> Kp1/1
  Kp4/1 -> Trigonometric Function1/1
  Selector/1 -> Variable Frequency Mean value/2  "Vq"
  2nd-Order Filter/1 -> Unit Delay/1
  Rate Limiter/1 -> 2nd-Order Filter/1
  Gain10/1 -> Rate Limiter/1
  Mux2/1 -> abc_to_dq0 Transformation/2, Sin_Cos/1
  Trigonometric Function2/1 -> Mux2/2
  Trigonometric Function/1 -> Mux2/1
  Math Function/1 -> theta/1, Trigonometric Function2/1, Trigonometric Function/1
  Constant4/1 -> Math Function/2
  abc_to_dq0 Transformation/1 -> Selector/1
  Vabc_pu/1 -> abc_to_dq0 Transformation/1

== system x35BusNetworkElectricityTransmissionModel/ 41.4 MW Wind Generation/41.4 MW Wind Farm/Control System/Control System 1/Measurement and abc-to-dq transformation /Discrete 3-phase PLL-Driven Positive-Sequence  ==
  note: Discrete 3-phase PLL-driven Positive-Sequence Active & Reactive Power
  note: Pierre Giroux, Gilbert Sybille
      | Power System Simulation Laboratory
      | IREQ, Hydro-Quebc
  wind_Freq : Inport  PortDimensions=1
  Sin_Cos : Inport  Port=2  PortDimensions=2
  Vabc_V : Inport  Port=3  PortDimensions=3
  Iabc_A : Inport  Port=4  PortDimensions=3
  Deg->Rad : Gain  Gain=pi/180  SaturateOnIntegerOverflow=on  OutDataTypeStr=Inherit: Same as input  ParamDataTypeStr=Inherit: Same as input
  Discrete 3-phase PLL-Driven Positive-Sequence Fundamental Value : Subsystem  mask(Discrete 3-phase PLL-Driven Positive-Sequence Fundamental Value){Finit=Finit, Fmin=Fmin, Par_Init=Par_Vinit, Ts=Ts}
      mask prompts: Finit "Initial frequency (Hz):"; Fmin "Minimum frequency (Hz):"; Par_Init "Initial input (positive component): [ Mag  Phase-relative-to-PLL(degrees) ]"; Ts "Sample time:"
      mask help:
      | For a supplied fundamental frequency (port Freq), this discrete block computes  the positive-sequence component (Magnitude and Phase)  of a set of three balanced or unbalanced signals (port abc) which may contain harmonics.
      |  Input port "Sin_Cos" (a two-dimension signal) provides the reference frame required for the computation..
      |  First and second outputs return respectively the magnitude and phase (in degrees relative to the PLL phase)) of the fundamental.
      | For the first cycle of simulation, the outputs are held constant to the values specified by the parameter "Initial input".
      | constant to the values specified by the parameter "Initial input". The value of the parameter "Minimum frequency" is used to determine the buffer size of the "Variable Transport Delay" block found inside this subsystem.
      mask init:
      | Real_Init=Par_Init(1)*cos(pi/180*Par_Init(2));
      | Imag_Init=Par_Init(1)*sin(pi/180*Par_Init(2));
      | power_initmask();
      settings: OpenFcn=power_openblockproxy();
  Discrete 3-phase PLL-Driven Positive-Sequence Fundamental Value2 : Subsystem  mask(Discrete 3-phase PLL-Driven Positive-Sequence Fundamental Value){Finit=Finit, Fmin=Fmin, Par_Init=Par_Iinit, Ts=Ts}
      mask prompts: Finit "Initial frequency (Hz):"; Fmin "Minimum frequency (Hz):"; Par_Init "Initial input (positive component): [ Mag  Phase-relative-to-PLL(degrees) ]"; Ts "Sample time:"
      mask help:
      | For a supplied fundamental frequency (port Freq), this discrete block computes  the positive-sequence component (Magnitude and Phase)  of a set of three balanced or unbalanced signals (port abc) which may contain harmonics.
      |  Input port "Sin_Cos" (a two-dimension signal) provides the reference frame required for the computation..
      |  First and second outputs return respectively the magnitude and phase (in degrees relative to the PLL phase)) of the fundamental.
      | For the first cycle of simulation, the outputs are held constant to the values specified by the parameter "Initial input".
      | constant to the values specified by the parameter "Initial input". The value of the parameter "Minimum frequency" is used to determine the buffer size of the "Variable Transport Delay" block found inside this subsystem.
      mask init:
      | Real_Init=Par_Init(1)*cos(pi/180*Par_Init(2));
      | Imag_Init=Par_Init(1)*sin(pi/180*Par_Init(2));
      | power_initmask();
      settings: OpenFcn=power_openblockproxy();
  Gain1 : Gain  Gain=3/2  SaturateOnIntegerOverflow=on  OutDataTypeStr=Inherit: Same as input  ParamDataTypeStr=Inherit: Same as input
  Gain2 : Gain  Gain=3/2  SaturateOnIntegerOverflow=on  OutDataTypeStr=Inherit: Same as input  ParamDataTypeStr=Inherit: Same as input
  Product : Product  InputSameDT=on  SaturateOnIntegerOverflow=on  OutDataTypeStr=Inherit: Same as first input
  Product1 : Product  InputSameDT=on  SaturateOnIntegerOverflow=on  OutDataTypeStr=Inherit: Same as first input
  Product2 : Product  InputSameDT=on  SaturateOnIntegerOverflow=on  OutDataTypeStr=Inherit: Same as first input
  Sum : Sum  Inputs=+-  InputSameDT=on  SaturateOnIntegerOverflow=on  OutDataTypeStr=Inherit: Same as first input
  Trigonometric Function : Trigonometry
  Trigonometric Function1 : Trigonometry  Operator=cos
  Mag_V_V : Outport  VectorParamsAs1DForOutWhenUnconnected=off
  P_W : Outport  Port=2  VectorParamsAs1DForOutWhenUnconnected=off
  Q_Var : Outport  Port=3  VectorParamsAs1DForOutWhenUnconnected=off
  wires:
  Vabc_V/1 -> Discrete 3-phase PLL-Driven Positive-Sequence Fundamental Value/3(abc)
  wind_Freq/1 -> Discrete 3-phase PLL-Driven Positive-Sequence Fundamental Value/1(Freq), Discrete 3-phase PLL-Driven Positive-Sequence Fundamental Value2/1(Freq)
  Sin_Cos/1 -> Discrete 3-phase PLL-Driven Positive-Sequence Fundamental Value/2(Sin_Cos), Discrete 3-phase PLL-Driven Positive-Sequence Fundamental Value2/2(Sin_Cos)
  Discrete 3-phase PLL-Driven Positive-Sequence Fundamental Value/2(Phase) -> Sum/1
  Discrete 3-phase PLL-Driven Positive-Sequence Fundamental Value/1(Mag) -> Product2/1, Mag_V_V/1
  Discrete 3-phase PLL-Driven Positive-Sequence Fundamental Value2/2(Phase) -> Sum/2
  Sum/1 -> Deg->Rad/1
  Deg->Rad/1 -> Trigonometric Function1/1, Trigonometric Function/1
  Trigonometric Function1/1 -> Product/2
  Trigonometric Function/1 -> Product1/1
  Product/1 -> Gain1/1
  Gain1/1 -> P_W/1
  Product2/1 -> Product/1, Product1/2
  Discrete 3-phase PLL-Driven Positive-Sequence Fundamental Value2/1(Mag) -> Product2/2
  Iabc_A/1 -> Discrete 3-phase PLL-Driven Positive-Sequence Fundamental Value2/3(abc)
  Product1/1 -> Gain2/1
  Gain2/1 -> Q_Var/1

== system x35BusNetworkElectricityTransmissionModel/ 41.4 MW Wind Generation/41.4 MW Wind Farm/Control System/Control System 1/Measurement and abc-to-dq transformation /Filter ==
  Vabc : Inport
  Stator_Iabc : Inport  Port=2
  Iabc_grid_conv : Inport  Port=3
  Rotor_Iabc : Inport  Port=4
  Vdc : Inport  Port=5
  Qref : Inport  Port=6
  wr : Inport  Port=7
  angle_rotor : Inport  Port=8
  Demux{,1..3} (4 alike) : Demux  Outputs=3
      settings: DisplayOption=none
  Discrete 2nd-Order Filter{1..6,8..16} (15 alike) : powerlib_extras/Discrete  Control Blocks/Discrete  2nd-Order Filter  FilterType=Lowpass  Fo=Freq  Zeta=Zeta1  Ts=Ts  Initialize=off  Vac_Init=[0.8 -25 60]  Vdc_Init=-0.4  PlotResponse=off  param1=[1 500 1]
  Discrete 2nd-Order Filter7 : powerlib_extras/Discrete  Control Blocks/Discrete  2nd-Order Filter  FilterType=Lowpass  Fo=Freq  Zeta=Zeta1  Ts=Ts  Initialize=on  Vac_Init=[0.8 -25 60]*0  Vdc_Init=wind_VDC_nom  PlotResponse=off  param1=[1 500 1]
  Mux{,1..3} (4 alike) : Mux  Inputs=3
  "Vabc " : Outport  VectorParamsAs1DForOutWhenUnconnected=off
  "Stator_Iabc " : Outport  Port=2  VectorParamsAs1DForOutWhenUnconnected=off
  "Iabc_grid_conv " : Outport  Port=3  VectorParamsAs1DForOutWhenUnconnected=off
  "Rotor_Iabc " : Outport  Port=4  VectorParamsAs1DForOutWhenUnconnected=off
  "Vdc " : Outport  Port=5  VectorParamsAs1DForOutWhenUnconnected=off
  "Qref " : Outport  Port=6  VectorParamsAs1DForOutWhenUnconnected=off
  "wr " : Outport  Port=7  VectorParamsAs1DForOutWhenUnconnected=off
  "angle_rotor " : Outport  Port=8  VectorParamsAs1DForOutWhenUnconnected=off
  wires:
  Demux/1 -> Discrete 2nd-Order Filter1/1
  Demux/2 -> Discrete 2nd-Order Filter2/1
  Demux/3 -> Discrete 2nd-Order Filter3/1
  Discrete 2nd-Order Filter1/1 -> Mux/1
  Discrete 2nd-Order Filter2/1 -> Mux/2
  Discrete 2nd-Order Filter3/1 -> Mux/3
  Vabc/1 -> Demux/1
  Mux/1 -> "Vabc "/1
  Demux1/1 -> Discrete 2nd-Order Filter5/1
  Demux1/2 -> Discrete 2nd-Order Filter6/1
  Demux1/3 -> Discrete 2nd-Order Filter4/1
  Discrete 2nd-Order Filter5/1 -> Mux1/1
  Discrete 2nd-Order Filter6/1 -> Mux1/2
  Discrete 2nd-Order Filter4/1 -> Mux1/3
  Iabc_grid_conv/1 -> Demux1/1
  Mux1/1 -> "Iabc_grid_conv "/1
  Vdc/1 -> Discrete 2nd-Order Filter7/1
  Discrete 2nd-Order Filter7/1 -> "Vdc "/1
  Demux2/1 -> Discrete 2nd-Order Filter8/1
  Demux2/2 -> Discrete 2nd-Order Filter9/1
  Demux2/3 -> Discrete 2nd-Order Filter10/1
  Discrete 2nd-Order Filter8/1 -> Mux2/1
  Discrete 2nd-Order Filter9/1 -> Mux2/2
  Discrete 2nd-Order Filter10/1 -> Mux2/3
  Stator_Iabc/1 -> Demux2/1
  Mux2/1 -> "Stator_Iabc "/1
  wr/1 -> Discrete 2nd-Order Filter13/1
  Discrete 2nd-Order Filter13/1 -> "wr "/1
  Demux3/1 -> Discrete 2nd-Order Filter15/1
  Demux3/2 -> Discrete 2nd-Order Filter16/1
  Demux3/3 -> Discrete 2nd-Order Filter14/1
  Discrete 2nd-Order Filter15/1 -> Mux3/1
  Discrete 2nd-Order Filter16/1 -> Mux3/2
  Discrete 2nd-Order Filter14/1 -> Mux3/3
  Rotor_Iabc/1 -> Demux3/1
  Mux3/1 -> "Rotor_Iabc "/1
  Qref/1 -> Discrete 2nd-Order Filter11/1
  Discrete 2nd-Order Filter11/1 -> "Qref "/1
  angle_rotor/1 -> Discrete 2nd-Order Filter12/1
  Discrete 2nd-Order Filter12/1 -> "angle_rotor "/1

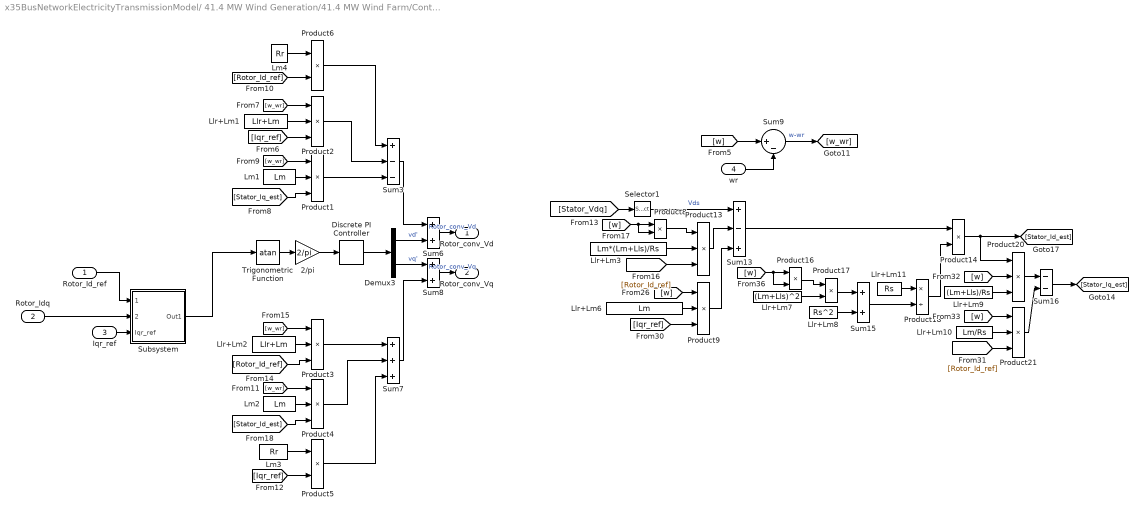
== system x35BusNetworkElectricityTransmissionModel/ 41.4 MW Wind Generation/41.4 MW Wind Farm/Control System/Control System 1/Rotor-side Control System/Current Regulator ==
  Rotor_Id_ref : Inport
  Rotor_Idq : Inport  Port=2
  Iqr_ref : Inport  Port=3
  wr : Inport  Port=4
  2/pi : Gain  Gain=2/pi
  Demux3 : Demux  Outputs=2
      settings: DisplayOption=none
  Discrete PI Controller : powerlib_extras/Discrete  Control Blocks/Discrete PI Controller  Kp=Rotor_Ireg_Kp  Ki=Rotor_Ireg_Ki  Par_Limits=[1 -1]* Rotor_Ireg_lim  Init=0  Ts=Ts
  Llr+Lm1 : Constant  Value=Llr+Lm
  Llr+Lm10 : Constant  Value=Lm/Rs
  Llr+Lm11 : Constant  Value=Rs
  Llr+Lm2 : Constant  Value=Llr+Lm
  Llr+Lm3 : Constant  Value=Lm*(Lm+Lls)/Rs
  Llr+Lm6 : Constant  Value=Lm
  Llr+Lm7 : Constant  Value=(Lm+Lls)^2
  Llr+Lm8 : Constant  Value=Rs^2
  Llr+Lm9 : Constant  Value=(Lm+Lls)/Rs
  Lm1 : Constant  Value=Lm
  Lm2 : Constant  Value=Lm
  Lm3 : Constant  Value=Rr
  Lm4 : Constant  Value=Rr  VectorParams1D=off
  Product{1..4,9,13,20..21} (8 alike) : Product  Inputs=3  SaturateOnIntegerOverflow=on  OutDataTypeStr=Inherit: Same as first input
  Product{5..6,8,14,16..17} (6 alike) : Product  SaturateOnIntegerOverflow=on  OutDataTypeStr=Inherit: Same as first input
  Product18 : Product  Inputs=*/  SaturateOnIntegerOverflow=on  OutDataTypeStr=Inherit: Same as first input
  Selector1 : Selector  InputPortWidth=2  IndexOptions=Index vector (dialog)  Indices=1  OutputSizes=[(-2)]
  Subsystem : Subsystem
  Sum13 : Sum  Inputs=+-+  InputSameDT=on  SaturateOnIntegerOverflow=on  OutDataTypeStr=Inherit: Same as first input
  Sum15 : Sum  InputSameDT=on  SaturateOnIntegerOverflow=on  OutDataTypeStr=Inherit: Same as first input
  Sum16 : Sum  Inputs=--  InputSameDT=on  SaturateOnIntegerOverflow=on  OutDataTypeStr=Inherit: Same as first input
  Sum3 : Sum  Inputs=+--  InputSameDT=on  SaturateOnIntegerOverflow=on  OutDataTypeStr=Inherit: Same as first input
  Sum6 : Sum  InputSameDT=on  SaturateOnIntegerOverflow=on  OutDataTypeStr=Inherit: Same as first input
  Sum7 : Sum  Inputs=+++  InputSameDT=on  SaturateOnIntegerOverflow=on  OutDataTypeStr=Inherit: Same as first input
  Sum8 : Sum  InputSameDT=on  SaturateOnIntegerOverflow=on  OutDataTypeStr=Inherit: Same as first input
  Sum9 : Sum  Inputs=|+-  InputSameDT=on  SaturateOnIntegerOverflow=on  OutDataTypeStr=Inherit: Same as first input
  Trigonometric Function : Trigonometry  Operator=atan
  Rotor_conv_Vd : Outport
  Rotor_conv_Vq : Outport  Port=2
  wires:
  Lm3/1 -> Product5/1
  Lm1/1 -> Product1/2
  Product8/1 -> Product13/1
  Sum8/1 -> Rotor_conv_Vq/1  "Rotor_conv_Vq"
  Selector1/1 -> Sum13/1  "Vds"
  Subsystem/1(Out1) -> Trigonometric Function/1
  Lm4/1 -> Product6/1
  Product13/1 -> Sum13/2
  Product6/1 -> Sum3/1
  Product1/1 -> Sum3/3
  Llr+Lm9/1 -> Product20/3
  Rotor_Idq/1 -> Subsystem/2(Rotor_Idq)
  Llr+Lm2/1 -> Product3/2
  Iqr_ref/1 -> Subsystem/3(Iqr_ref)
  [w_wr] -> Product4/1
  Product18/1 -> Product14/2
  [w] -> Product20/2
  Sum3/1 -> Sum6/1
  Sum15/1 -> Product18/2
  Sum7/1 -> Sum8/2
  [w] -> Product16/2, Product16/1
  [Rotor_Id_ref] -> Product6/2
  [w_wr] -> Product1/1
  Llr+Lm3/1 -> Product13/2
  Product21/1 -> Sum16/2
  [Iqr_ref] -> Product9/3
  [w_wr] -> Product3/1
  Product4/1 -> Sum7/2
  Product17/1 -> Sum15/1
  Llr+Lm11/1 -> Product18/1
  Demux3/2 -> Sum8/1  "vq'"
  [Stator_Id_est] -> Product4/3
  Product14/1 -> [Stator_Id_est], Product20/1
  [Rotor_Id_ref] -> Product21/3
  [Stator_Vdq] -> Selector1/1
  Sum16/1 -> [Stator_Iq_est]
  Llr+Lm8/1 -> Sum15/2
  Demux3/1 -> Sum6/2  "vd'"
  Lm2/1 -> Product4/2
  Product20/1 -> Sum16/1
  [w_wr] -> Product2/1
  [w] -> Product9/1
  Llr+Lm7/1 -> Product17/2
  [Iqr_ref] -> Product5/2
  Trigonometric Function/1 -> 2/pi/1
  Sum13/1 -> Product14/1
  [Rotor_Id_ref] -> Product3/3
  Llr+Lm1/1 -> Product2/2
  [Rotor_Id_ref] -> Product13/3
  Product5/1 -> Sum7/3
  [w] -> Sum9/1
  Sum9/1 -> [w_wr]  "w-wr"
  Discrete PI Controller/1 -> Demux3/1
  wr/1 -> Sum9/2
  Product9/1 -> Sum13/3
  [w] -> Product8/1, Product8/2
  Llr+Lm10/1 -> Product21/2
  2/pi/1 -> Discrete PI Controller/1
  [Stator_Iq_est] -> Product1/3
  [Iqr_ref] -> Product2/3
  Product3/1 -> Sum7/1
  Product16/1 -> Product17/1
  Llr+Lm6/1 -> Product9/2
  Product2/1 -> Sum3/2
  [w] -> Product21/1
  Rotor_Id_ref/1 -> Subsystem/1(Rotor_Id_ref)
  Sum6/1 -> Rotor_conv_Vd/1  "Rotor_conv_Vd"

== system x35BusNetworkElectricityTransmissionModel/ 41.4 MW Wind Generation/41.4 MW Wind Farm/Control System/Control System 1/Rotor-side Control System/Electromagnetic Torque Controller  ==
  Stator_Vdq : Inport
  w : Inport  Port=2
  Stator_Idq : Inport  Port=3
  Tem_cmd : Inport  Port=4
  Divide2 : Product  Inputs=*/
  Divide3 : Product  Inputs=**
  Lm/Ls : Constant  Value=Lm/(Lls+Lm)
  Min_flux-inf : Saturate  UpperLimit=inf  LowerLimit=Flux_min
  Saturation : Saturate  UpperLimit=Idref_max  LowerLimit=0
  Stator flux estimator : Subsystem
  Rotor_Id_ref : Outport
  wires:
  Stator_Idq/1 -> Stator flux estimator/2(Stator_Idq), [Stator_Idq]
  Lm/Ls/1 -> Divide3/2
  Stator flux estimator/1(Mag_Flux) -> Min_flux-inf/1
  Divide2/1 -> Saturation/1
  w/1 -> Stator flux estimator/3(w_pu), [w]
  Min_flux-inf/1 -> Divide3/1
  Saturation/1 -> Rotor_Id_ref/1
  Stator_Vdq/1 -> [Stator_Vdq], Stator flux estimator/1(Stator_Vdq)
  Divide3/1 -> Divide2/2
  Tem_cmd/1 -> Divide2/1

== system x35BusNetworkElectricityTransmissionModel/ 41.4 MW Wind Generation/41.4 MW Wind Farm/Control System/Control System 1/Rotor-side Control System/Iqr, ref_limit ==
  Rotor_Id_ref : Inport
  Constant1 : Constant
  Constant4 : Constant
  Demux4 : Demux  Outputs=2
      settings: DisplayOption=none
  Discrete-Time Integrator2 : DiscreteIntegrator  gainval=10  SampleTime=Ts  LimitOutput=on  UpperSaturationLimit=1  LowerSaturationLimit=0  ICPrevOutput=DiscIntNeverNeededParam  ICPrevScaledInput=DiscIntNeverNeededParam
  Divide1 : Product  Inputs=**
  Irotor_max^2 : Constant
  Math Function : Math  Operator=square  SignedPower=on
  Math Function1 : Math  Operator=sqrt  SignedPower=on
  Math Function2 : Math  Operator=square  SignedPower=on
  Math Function3 : Math  Operator=square  SignedPower=on
  Math Function4 : Math  Operator=sqrt  SignedPower=on
  Sum1 : Sum  Inputs=|-+  InputSameDT=on  SaturateOnIntegerOverflow=on  OutDataTypeStr=Inherit: Same as first input
  Sum10 : Sum  Inputs=|++  InputSameDT=on  SaturateOnIntegerOverflow=on  OutDataTypeStr=Inherit: Same as first input
  Sum11 : Sum  Inputs=|+-  InputSameDT=on  SaturateOnIntegerOverflow=on  OutDataTypeStr=Inherit: Same as first input
  Sum12 : Sum  Inputs=|+-  InputSameDT=on  SaturateOnIntegerOverflow=on  OutDataTypeStr=Inherit: Same as first input
  t=Iq_ref_limit_time_constants : powerlib_extras/Discrete  Control Blocks/Discrete 1st-Order Filter  FilterType=Lowpass  Tc=Iqref_Tc  Ts=Ts  Initialize=on  Vac_Init=[0 0 0]  Vdc_Init=Grid_conv_Imax  PlotResponse=off  param1=[1 500 0.1]
  Iqrlim : Outport
  wires:
  Discrete-Time Integrator2/1 -> Sum12/2
  Sum12/1 -> Divide1/2
  Demux4/2 -> Math Function3/1
  Math Function3/1 -> Sum10/2
  Math Function2/1 -> Sum10/1
  Math Function1/1 -> t=Iq_ref_limit_time_constants/1
  t=Iq_ref_limit_time_constants/1 -> Divide1/1
  Demux4/1 -> Math Function2/1
  Constant1/1 -> Sum11/2
  Constant4/1 -> Sum12/1
  Sum11/1 -> Discrete-Time Integrator2/1
  Math Function/1 -> Sum1/1
  [Stator_Idq] -> Demux4/1
  Sum10/1 -> Math Function4/1
  Irotor_max^2/1 -> Sum1/2
  Rotor_Id_ref/1 -> Math Function/1
  Sum1/1 -> Math Function1/1
  Divide1/1 -> Iqrlim/1  "Iqrlim"
  Math Function4/1 -> Sum11/1

== system x35BusNetworkElectricityTransmissionModel/ 41.4 MW Wind Generation/41.4 MW Wind Farm/Control System/Control System 1/Rotor-side Control System/Modulation Index & Phase ==
  note: m = Vnom_r * 2*sqrt(2/3) / Vdc
  note: Required value for modulation index "m" to obtain 1 pu generated voltage by the converter:
  note: Where Vnom_r = RMS ph-ph nominal voltage
  x : Inport
  y : Inport  Port=2
  Vdc : Inport  Port=3
  0-Mod_index_max_rotor : Saturate  UpperLimit=Rotor_Modindex_Upper  LowerLimit=0
  Avoid division by zero : Saturate  UpperLimit=inf  LowerLimit=1e-6
  Cartesian to Polar : simulink_extras/Transformations/Cartesian to Polar
  K : Constant  Value=Wind_Rotor_V_nom*2*sqrt(2/3)
  Polar to Cartesian : simulink_extras/Transformations/Polar to Cartesian
  Product7 : Product  Inputs=**/  InputSameDT=on  SaturateOnIntegerOverflow=on  OutDataTypeStr=Inherit: Same as first input
  x1 : Outport
  y1 : Outport  Port=2
  wires:
  Vdc/1 -> Avoid division by zero/1
  Product7/1 -> 0-Mod_index_max_rotor/1  "m"
  Polar to Cartesian/1 -> x1/1
  Cartesian to Polar/1 -> Product7/1
  Cartesian to Polar/2 -> Polar to Cartesian/2
  K/1 -> Product7/2
  0-Mod_index_max_rotor/1 -> Polar to Cartesian/1
  Avoid division by zero/1 -> Product7/3
  Polar to Cartesian/2 -> y1/1
  x/1 -> Cartesian to Polar/1
  y/1 -> Cartesian to Polar/2

== system x35BusNetworkElectricityTransmissionModel/ 41.4 MW Wind Generation/41.4 MW Wind Farm/Control System/Control System 1/Rotor-side Control System/Rotor Control Voltage Converter ==
  x1 : Inport
  y1 : Inport  Port=2
  Angle : Inport  Port=3
  Mux4 : Mux  Inputs=3
  Mux5 : Mux  Inputs=2
  Trigonometric Function2 : Trigonometry
  Trigonometric Function3 : Trigonometry  Operator=cos
  V0 : Constant  Value=0
  dq0_to_abc Transformation : powerlib_extras/Measurements/dq0_to_abc Transformation
  Uctrl_rotor_conv : Outport  VectorParamsAs1DForOutWhenUnconnected=off
  wires:
  Mux5/1 -> dq0_to_abc Transformation/2
  Trigonometric Function2/1 -> Mux5/1
  Mux4/1 -> dq0_to_abc Transformation/1  "Vdq0"
  Trigonometric Function3/1 -> Mux5/2
  Angle/1 -> Trigonometric Function3/1, Trigonometric Function2/1
  dq0_to_abc Transformation/1 -> Uctrl_rotor_conv/1
  V0/1 -> Mux4/3
  x1/1 -> Mux4/1
  y1/1 -> Mux4/2
